simulink model "modelo_BDA"  (R2021b)
settings: Solver=ode3  StartTime=0.0  StopTime=10.0  FixedStep=1e-6  RelTol=1e-3
(part 1 of 4)
settings Model: Creator=Alejandro TeveraRuiz  LastModifiedBy=Alejandro TeveraRuiz

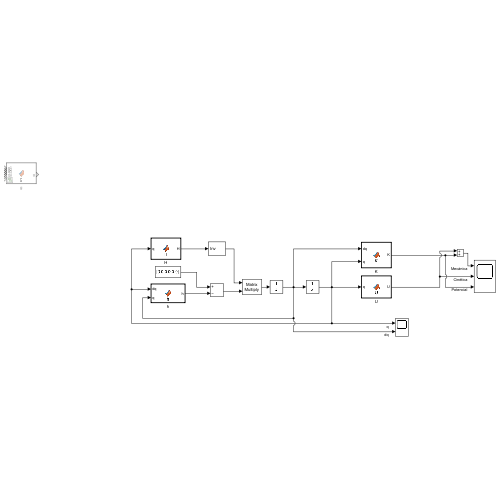
[thumbnail: Simulink's stored preview of the top-level diagram]
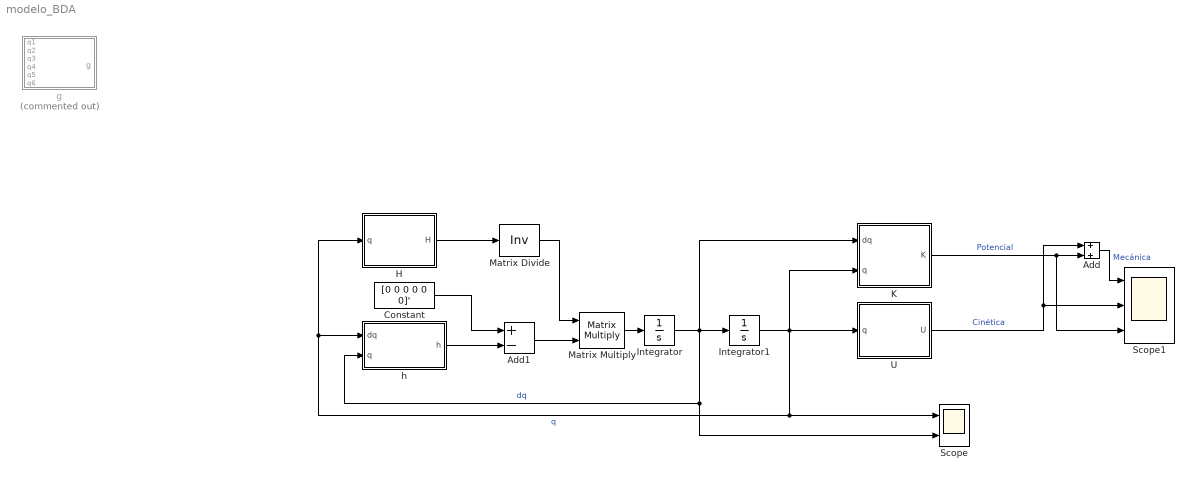
== system modelo_BDA ==
  Add : Sum
  Add1 : Sum  Inputs=+-
  Constant : Constant  Value=[0 0 0 0 0 0]'
  H : MATLAB Function  TreatAsAtomicUnit=on
  Integrator : Integrator  InitialCondition=[0 0 0 0 0 0]'
  Integrator1 : Integrator  InitialCondition=[0 0 0 0 0 0]'
  K : MATLAB Function  TreatAsAtomicUnit=on
  Matrix Divide : Product  Inputs=/  Multiplication=Matrix(*)  OutDataTypeStr=double
  Matrix Multiply : Product  Multiplication=Matrix(*)  OutDataTypeStr=double
  Scope : Scope  NumInputPorts=2
  Scope1 : Scope  NumInputPorts=3
  U : MATLAB Function  TreatAsAtomicUnit=on
  g : MATLAB Function  Commented=on  TreatAsAtomicUnit=on
  h : MATLAB Function  TreatAsAtomicUnit=on
  wires:
  Integrator/1 -> K/1(dq), Scope/2, h/2(q), Integrator1/1  "dq"
  Constant/1 -> Add1/1
  K/1(K) -> Add/2, Scope1/3  "Potencial"
  U/1(U) -> Add/1, Scope1/2  "Cinética"
  Add/1 -> Scope1/1  "Mecánica"
  h/1(h) -> Add1/2
  H/1(H) -> Matrix Divide/1
  Integrator1/1 -> K/2(q), U/1(q), H/1(q), h/1(dq), Scope/1  "q"
  Matrix Multiply/1 -> Integrator/1
  Matrix Divide/1 -> Matrix Multiply/1
  Add1/1 -> Matrix Multiply/2

== matlab function modelo_BDA/H ==
  data: q input; H output
function H = H(q)
%#codegen
q2 = q(2);
q3 = q(3);
q4 = q(4);
q5 = q(5);
q6 = q(6);
%    This function was generated by the Symbolic Math Toolbox version 9.0.
%    01-Dec-2021 19:55:30

t2 = cos(q2);
t3 = cos(q4);
t4 = cos(q5);
t5 = cos(q6);
t6 = sin(q2);
t7 = sin(q4);
t8 = sin(q5);
t9 = sin(q6);
t19 = 9.007199254740992e+15;
t10 = t2.*3.235524933e+1;
t11 = t6.*3.235524933e+1;
t12 = t2.*1.0513390433e+2;
t13 = t6.*1.0513390433e+2;
t14 = t4.*5.110348748545983e-1;
t16 = t8.*5.110348748545983e-1;
t17 = t5.*t8.*4.360410618e+1;
t18 = t8.*t9.*4.360410618e+1;
t20 = t3.*5.157359871151559;
t21 = t4.*t7.*8.595599785252598e-1;
t22 = t3.*t9.*8.595599785252598e-1;
t23 = t7.*t8.*8.595599785252598e-1;
t24 = t3.*t5.*8.595599785252598e-1;
t26 = (q3.*t19)./9.007199254740992e+15;
t29 = q3.*t19.*1.110223024625157e-16i;
t36 = t8.*7.263507131821755e+1;
t37 = t9.*7.263507131821755e+1;
t38 = t5.*1.336375981993753e+2;
t39 = t8.*1.336375981993753e+2;
t42 = t4.*1.356524863046341e+2;
t43 = t3.*3.748034457169395e+1;
t44 = t4.*t9.*1.336375981993753e+2;
t45 = t8.*6.185536839278779e+1;
t46 = t4.*t5.*7.263507131821755e+1;
t47 = t5.*t8.*8.018255891962515e+2;
t50 = t8.*t9.*4.358104279093053e+2;
t51 = t3.*t4.*4.931128922368695e+1;
t52 = t5.*t7.*4.931128922368695e+1;
t53 = t7.*t9.*4.931128922368695e+1;
t54 = t4.*t5.*1.40259874879e-5;
t55 = t4.*t9.*1.40259874879e-5;
t57 = t3.*t8.*t9.*4.931128922368695e+1;
t58 = t5.*t8.*8.415592492740001e-5;
t59 = t8.*t9.*8.415592492740001e-5;
t61 = t3.*t5.*t8.*4.931128922368695e+1;
t71 = t3.*9.473039288601392e+2;
t72 = t7.*9.473039288601392e+2;
t76 = t4.*7.291450524218959e+2;
t77 = t8.*7.291450524218959e+2;
t79 = t5.*1.246862890394724e+3;
t80 = t9.*1.246862890394724e+3;
t82 = t2.*1.908064859676306e+4;
t83 = t8.*6.829347327168682e+1;
t85 = t8.*3.711905458116013e+1;
t86 = t3.*6.892171862305337e+2;
t87 = t8.*4.200920957332826e+3;
t89 = t6.*5.850608528728732e+4;
t90 = t3.*3.746052020548068e+2;
t91 = t3.*5.316839912737671e+1;
t94 = t4.*6.932315136240378e+1;
t95 = t8.*3.161025044569338e+1;
t97 = t4.*t7.*6.243420034246779e+1;
t98 = t3.*t9.*6.243420034246779e+1;
t99 = t5.*t7.*3.583624485303893e+2;
t100 = t7.*t9.*3.583624485303893e+2;
t101 = t4.*2.524704765397172;
t102 = t4.*t5.*(-1.246862890394724e+3);
t103 = t7.*1.451748464558917e+2;
t104 = t4.*t9.*(-1.246862890394724e+3);
t105 = t3.*1.166014482149094e+2;
t106 = t3.*t5.*1.148695310384223e+2;
t107 = t4.*t7.*1.148695310384223e+2;
t109 = t3.*t4.*3.583624485303893e+2;
t110 = t8.*3.603346018435275e-1;
t111 = t4.*t7.*5.316839912737671e+1;
t112 = t7.*5.363537921262857e+2;
t113 = t8.*1.758766552463174e+1;
t114 = t4.*3.603346018435275e-1;
t116 = t5.*3.146556876441599e-4;
t117 = t8.*3.146556876441599e-4;
t118 = t7.*t8.*1.166014482149094e+2;
t119 = t3.*t5.*t8.*3.583624485303893e+2;
t120 = t8.*4.126305645247942e-4;
t121 = t9.*4.126305645247942e-4;
t122 = t3.*t8.*t9.*3.583624485303893e+2;
t124 = t3.*1.607982057580514e-1;
t126 = t3.*t4.*5.363537921262857e+2;
t127 = t3.*t8.*5.363537921262857e+2;
t130 = t4.*t7.*6.060823201364798e-1;
t131 = t4.*t9.*3.146556876441599e-4;
t132 = t7.*t8.*6.060823201364798e-1;
t133 = t4.*t5.*4.126305645247942e-4;
t135 = t3.*t5.*1.205617750389489e-5;
t136 = t3.*t9.*1.205617750389489e-5;
t138 = t8.*5.878411097842592e+2;
t140 = t4.*2.257319383180457e+3;
t144 = t5.*3.383303336574349e+3;
t145 = t9.*1.744166601788531e+3;
t147 = t4.*t5.*1.744166601788531e+3;
t148 = t4.*t9.*3.383303336574349e+3;
t156 = t3.*2.748657914322168e+3;
t164 = t4.*3.726185506152731e+2;
t165 = t8.*3.726185506152731e+2;
t166 = t3.*2.286243086622337e+3;
t167 = t8.*2.14681711570464e+3;
t168 = t7.*6.685860485757689;
t171 = t7.*3.050167960854463e+3;
t172 = t7.*6.689198986080043e+3;
t176 = t3.*t4.*3.581729009555754e+3;
t177 = t7.*t9.*3.581729009555754e+3;
t178 = t4.*t7.*3.610943527871318e+3;
t179 = t4.*t7.*6.267439056015643e+2;
t180 = t3.*t5.*1.071753439291633e+3;
t181 = t7.*t8.*6.267439056015643e+2;
t182 = t3.*t9.*1.071753439291633e+3;
t183 = t3.*t4.*6.589842255968259e+3;
t186 = t5.*t7.*6.589842255968259e+3;
t187 = t7.*3.119613856461354e+4;
t188 = t3.*t4.*3.050167960854463e+3;
t190 = t3.*2.170135173927414;
t192 = t3.*t8.*6.689198986080043e+3;
t193 = t8.*2.108686089031105e-4;
t194 = t8.*8.987910450364716;
t195 = t4.*1.290212183829552;
t196 = t3.*1.511765340066191e+1;
t198 = t3.*t8.*t9.*6.589842255968259e+3;
t201 = t3.*t5.*t8.*3.581729009555754e+3;
t203 = t8.*1.608000299575208e-4;
t204 = t7.*t8.*2.170135173927414;
t205 = t3.*1.454828146091616;
t206 = t7.*1.454828146091616;
t208 = t3.*t4.*3.476976747206118e+1;
t209 = t3.*t8.*3.476976747206118e+1;
t211 = t4.*t7.*1.511765340066191e+1;
t213 = t4.*t7.*3.54680719181798e-4;
t214 = t3.*t9.*3.54680719181798e-4;
t216 = t3.*t5.*2.704654361142649e-4;
t217 = t5.*t7.*6.916395256636513e-4;
t218 = t4.*t7.*2.704654361142649e-4;
t219 = t7.*t9.*6.916395256636513e-4;
t223 = t8.*3.004073079729871e+2;
t224 = t3.*t5.*t8.*6.916395256636513e-4;
t225 = t3.*t8.*t9.*6.916395256636513e-4;
t227 = t4.*1.153568928490484e+3;
t229 = t7.*t8.*1.940301400531246e+3;
t230 = t4.*t7.*5.052846917024227e+2;
t235 = t3.*2.862617746347316e+4;
t249 = t3.*t5.*2.908152143330287e+3;
t250 = t3.*t9.*1.499215806777825e+3;
t15 = -t13;
t25 = -t23;
t27 = cos(t26);
t28 = sin(t26);
t30 = exp(t29);
t31 = -t29;
t48 = -t44;
t49 = -t45;
t56 = t11+t12;
t62 = -t61;
t63 = t16+t21;
t84 = -t77;
t92 = t4.*t79;
t93 = t4.*t80;
t96 = -t90;
t108 = -t94;
t115 = -t110;
t123 = -t114;
t125 = -t116;
t128 = -t119;
t129 = -t121;
t134 = -t130;
t137 = -t136;
t139 = -t138;
t141 = t20+t51;
t161 = -t156;
t169 = -t164;
t189 = -t176;
t191 = -t180;
t197 = -t192;
t199 = -t194;
t200 = -t195;
t202 = -t196;
t207 = -t201;
t210 = -t204;
t215 = -t209;
t221 = -t211;
t222 = -t214;
t226 = -t224;
t228 = -t227;
t253 = -t250;
t275 = t37+t38+4.360410618e+1;
t280 = t18+t36+t55;
t282 = t17+t39+t54;
t303 = t71-8.631091645042425e+1;
t304 = t72+9.559948463095517e-2;
t311 = t101+t113;
t312 = t103+t124;
t443 = t79+t145+4.358104279093053e+2;
t446 = t80+t144+8.018255891962515e+2;
t531 = t187+t205+2.538346896821816;
t532 = t58+t104+t120+t147;
t533 = t59+t102+t117+t148;
t537 = t206+t235-3.371409213983255e+2;
t556 = t47+t50+t87+t131+t133;
t32 = 1.0./t30;
t33 = t3.*t27;
t34 = t7.*t27;
t40 = t30-1.0;
t60 = t10+t15;
t64 = t14+t25;
t66 = t5.*t63.*6.0;
t68 = t9.*t63.*6.0;
t70 = t27.*1.318958611e+1;
t142 = t5.*t63.*4.360410618e+1;
t143 = t9.*t63.*4.360410618e+1;
t150 = t27.*3.811321279694577e+2;
t151 = t27.*3.422984996757468e+1;
t155 = t27.*3.079131064925427e+1;
t170 = t30.*3.694216783411725e-1;
t173 = t30.*1.305783216588275e-1;
t212 = t42+t49;
t220 = t46+t48;
t232 = t9.*t63.*4.358104279093053e+2;
t234 = t5.*t63.*8.018255891962515e+2;
t237 = t5.*t63.*8.415592492740001e-5;
t238 = t9.*t63.*8.415592492740001e-5;
t241 = t3.*t19.*t28.*5.673626844500105e-17;
t242 = t7.*t19.*t28.*5.673626844500105e-17;
t243 = t4.*t19.*t28.*9.543032792050485e-17;
t244 = t8.*t19.*t28.*9.543032792050485e-17;
t245 = t3.*t19.*t28.*3.404176106700063e-16;
t248 = t27.*2.227646919556693e+3;
t252 = t27.*8.579529175625027e+2;
t256 = t27.*2.467380792691235;
t259 = t30.*3.269483204543573;
t264 = t30.*1.334999662191606e+1;
t271 = t27.*1.104616756676389e-4;
t272 = t27.*5.202289239433555e-4;
t285 = t3.*t19.*t28.*2.556183965391409e-15;
t286 = t7.*t19.*t28.*2.556183965391409e-15;
t287 = t19.*t28.*4.869208971920574e-15;
t288 = t7.*t19.*t28.*9.827649182848514e-15;
t289 = t3.*t19.*t28.*2.473934273532809e-15;
t292 = t7.*t19.*t28.*4.958440210927941e-15;
t293 = t7.*t19.*t28.*7.425392937311983e-15;
t295 = t3.*t19.*t28.*7.425392937311983e-15;
t297 = t30.*3.857674212413887e+2;
t299 = t30.*1.091297471081935e+1;
t305 = t30.*4.456000120203464e+1;
t306 = t27.*3.608035586078749e-4;
t313 = t121+t125;
t314 = t116+t129;
t315 = t76+t139;
t316 = t84+t140;
t317 = t8.*t19.*t28.*1.275307981867505e-14;
t318 = t3.*t19.*t28.*4.549259187470966e-14;
t319 = t19.*t28.*1.611764571317528e-14;
t320 = t3.*t19.*t28.*1.117556177536684e-13;
t321 = t7.*t19.*t28.*1.117556177536684e-13;
t323 = t3.*t19.*t28.*2.524584390187751e-13;
t324 = t7.*t19.*t28.*2.524584390187751e-13;
t325 = t7.*t19.*t28.*1.068943235898118e-13;
t326 = t3.*t19.*t28.*7.696415878211547e-15;
t327 = t7.*t19.*t28.*5.39324412732078e-14;
t328 = t4.*t19.*t28.*1.294536125128302e-14;
t330 = t7.*t19.*t28.*9.582436671975919e-15;
t331 = t8.*t19.*t28.*6.931588674426758e-15;
t332 = t3.*t19.*t28.*2.472625742899312e-14;
t335 = t19.*t28.*1.78521870351002e-17;
t338 = t3.*t19.*t28.*3.509442785897641e-15;
t340 = t8.*t19.*t28.*5.90287808936737e-15;
t341 = t3.*t19.*t28.*1.061367489795852e-17;
t342 = t19.*t28.*2.126613508315838e-14;
t345 = t4.*t19.*t28.*6.72886546633755e-17;
t346 = t8.*t19.*t28.*6.72886546633755e-17;
t347 = t19.*t28.*9.790736217417458e-22;
t349 = t19.*t28.*1.646800527103812e-21;
t356 = t30.*2.254739352916933e+3;
t357 = t19.*t28.*t56.*5.673626844500105e-17;
t360 = t30.*2.497388846980927;
t362 = t30.*5.576400544494359e+2;
t365 = t30.*5.642007925493603e-5;
t371 = t30.*2.303752062145191e-4;
t373 = t19.*t28.*6.295748150968656e-14;
t374 = t7.*t19.*t28.*3.067061459005602e-13;
t375 = t7.*t19.*t28.*6.726247428052494e-13;
t376 = t7.*t19.*t28.*6.078928606401748e-13;
t378 = t7.*t19.*t28.*1.333145046183106e-12;
t380 = t4.*t19.*t28.*6.958255145423523e-14;
t381 = t8.*t19.*t28.*4.008952645263927e-13;
t382 = t8.*t19.*t28.*6.958255145423523e-14;
t384 = t3.*t19.*t28.*1.509061667990639e-13;
t385 = t3.*t19.*t28.*1.657497724402608e-13;
t389 = t3.*t19.*t28.*4.691552578623493e-13;
t390 = t3.*t19.*t28.*1.291537270195008e-12;
t391 = t19.*t28.*4.740092871521216e-16;
t392 = t8.*t19.*t28.*1.678396688371765e-15;
t393 = t3.*t19.*t28.*1.432423273139473e-16;
t394 = t3.*t19.*t28.*9.978585125263967e-16;
t395 = t4.*t19.*t28.*2.409334036643134e-16;
t396 = t7.*t19.*t28.*7.599994046755678e-16;
t398 = t3.*t19.*t28.*9.602764472540121e-17;
t399 = t8.*t19.*t28.*3.002769545393412e-20;
t400 = t7.*t19.*t28.*9.602764472540121e-17;
t401 = t7.*t19.*t28.*6.448744418276857e-12;
t402 = t7.*t19.*t28.*3.19687103847679e-12;
t403 = t19.*t28.*4.337843352208199e-20;
t410 = t7.*t19.*t28.*1.670884143038041e-15;
t411 = t8.*t19.*t28.*3.937747008262415e-20;
t416 = t8.*t19.*t28.*5.609786987186535e-14;
t417 = t19.*t28.*3.910962660750154e-13;
t418 = t4.*t19.*t28.*2.154167289582227e-13;
t419 = t19.*t28.*t56.*1.893759423098155e-16;
t423 = t3.*t19.*t28.*3.027237730074418e-12;
t425 = t3.*t19.*t28.*6.279111109874485e-12;
t430 = t30.*2.268539354478371e-4;
t432 = t19.*t28.*2.007862416620223e-13;
t433 = t19.*t28.*2.261065882456945e-13;
t438 = t19.*t28.*5.703946554323684e-14;
t452 = t19.*t28.*t56.*1.74698406676951e-15;
t454 = t19.*t28.*t56.*1.942073956592427e-15;
t459 = t19.*t28.*1.428243658465093e-13;
t491 = t19.*t28.*t56.*5.091700655507849e-16;
t530 = t161+t168+2.094342917444822e+3;
t540 = t91+t123+t126+t132;
t541 = t105+t115+t127+t134;
t585 = t95+t108+t111+t112+t118;
t665 = t166+t188+t192+t199+t200+t204+t221;
t666 = t165+t172+t179+t190+t208+t228+t229;
t667 = t169+t171+t181+t202+t215+t223+t230;
t35 = t34.*6.0;
t41 = t40.^2;
t65 = t5.*t64;
t67 = t9.*t64;
t73 = t34.*4.360410618e+1;
t74 = t33.*2.286892447e+1;
t75 = t34.*2.286892447e+1;
t81 = t33.*6.520967601e+1;
t152 = t34.*4.358104279093053e+2;
t153 = t33.*1.328674864713371e+3;
t154 = t34.*1.328674864713371e+3;
t157 = t34.*8.018255891962515e+2;
t158 = t34.*6.185536839278779e+1;
t159 = t33.*1.688943762888624e+2;
t160 = t34.*1.356524863046341e+2;
t163 = t33.*7.092789006718835e+2;
t174 = t34.*1.870703729528352e-1;
t175 = t32.*3.694216783411725e-1;
t184 = t32.*1.305783216588275e-1;
t246 = -t242;
t247 = -t243;
t251 = t34.*4.522154679359383e+3;
t254 = t34.*2.65978307941329e+3;
t255 = t34.*2.92140771649329e+3;
t257 = t33.*4.033568532372886e+3;
t258 = t33.*8.84585468187615e+3;
t261 = t33.*9.245169992678717;
t262 = t32.*3.269483204543573;
t263 = t34.*2.524704765397172;
t266 = t33.*4.153012702745543e+4;
t267 = t34.*1.758766552463174e+1;
t268 = t32.*1.334999662191606e+1;
t269 = t33.*1.692526621106363;
t270 = t34.*1.692526621106363;
t274 = -t271;
t276 = -t272;
t277 = t34.*3.854027039691565e+4;
t294 = -t288;
t296 = -t293;
t298 = t34.*2.310978750639558e+3;
t300 = t32.*3.857674212413887e+2;
t301 = t32.*1.091297471081935e+1;
t302 = t33.*4.724604290218056;
t307 = t32.*4.456000120203464e+1;
t308 = -t306;
t322 = -t318;
t329 = -t321;
t333 = -t324;
t334 = -t325;
t336 = -t327;
t337 = -t328;
t339 = -t330;
t343 = -t341;
t344 = t34+t241;
t350 = -t347;
t358 = t32.*2.254739352916933e+3;
t359 = t19.*t28.*t60.*9.543032792050485e-17;
t363 = t32.*2.497388846980927;
t364 = t32.*5.576400544494359e+2;
t366 = t32.*5.642007925493603e-5;
t368 = t52+t57+t66;
t369 = t53+t62+t68;
t372 = t32.*2.303752062145191e-4;
t377 = -t373;
t379 = -t374;
t383 = -t376;
t386 = -t378;
t387 = -t380;
t388 = -t382;
t397 = -t393;
t404 = -t396;
t405 = -t398;
t406 = -t399;
t407 = -t400;
t408 = -t401;
t409 = -t402;
t412 = -t403;
t413 = -t410;
t420 = -t418;
t421 = t19.*t28.*t60.*3.18530082611956e-16;
t424 = -t423;
t427 = -t425;
t431 = t32.*2.268539354478371e-4;
t434 = -t432;
t439 = -t438;
t455 = -t452;
t457 = t19.*t28.*t60.*2.938424872360468e-15;
t461 = t19.*t28.*t60.*3.266565807075334e-15;
t493 = -t491;
t497 = t19.*t28.*t60.*8.564233717611997e-16;
t589 = t19.*t28.*t530.*9.543032792050485e-17;
t69 = -t65;
t78 = -t74;
t88 = -t81;
t146 = t24+t67;
t162 = -t157;
t185 = -t174;
t231 = t67.*1.336375981993753e+2;
t233 = t65.*7.263507131821755e+1;
t239 = t65.*1.40259874879e-5;
t240 = t67.*1.40259874879e-5;
t260 = -t258;
t265 = -t263;
t273 = -t270;
t278 = -t277;
t279 = t65.*1.246862890394724e+3;
t281 = t67.*1.246862890394724e+3;
t290 = t65.*4.126305645247942e-4;
t291 = t67.*3.146556876441599e-4;
t309 = t65.*1.744166601788531e+3;
t310 = t67.*3.383303336574349e+3;
t348 = t33+t246;
t351 = t5.*t344;
t352 = t9.*t344;
t361 = -t359;
t367 = t32.*t41.*5.499266393288274;
t370 = t32.*t41.*7.936984065608979;
t414 = t4.*t344.*4.234075154e+1;
t415 = t8.*t344.*4.234075154e+1;
t422 = -t421;
t426 = t32.*t41.*1.589092398552061e+2;
t428 = t32.*t41.*1.835560892149977e+1;
t429 = t32.*t41.*2.649229280878313e+1;
t435 = t32.*t41.*t56.*2.196325630278387e-1;
t436 = t32.*t41.*t60.*2.196325630278387e-1;
t440 = t4.*t344.*3.077051043151931e+2;
t441 = t37.*t344;
t442 = t38.*t344;
t448 = t4.*t344.*4.605359747732407e+2;
t450 = t8.*t344.*4.605359747732407e+2;
t465 = -t461;
t466 = t32.*t41.*9.287951675407251e+2;
t467 = t32.*t41.*1.02874981515943;
t468 = t32.*t41.*4.326292055563303e+2;
t469 = t32.*t41.*1.369651538214088e-4;
t470 = t32.*t41.*9.489849812415379e-5;
t471 = t32.*t41.*t56.*6.34659991754557;
t472 = t32.*t41.*t56.*7.330958613472507e-1;
t473 = t32.*t41.*t60.*7.330958613472507e-1;
t475 = t4.*t344.*5.658316341762099e+3;
t476 = t4.*t344.*3.07542350777483e+3;
t477 = t4.*t344.*2.619002784534197e+3;
t478 = t4.*t344.*4.465233410425356e+3;
t479 = t8.*t344.*5.743628218407764e+3;
t480 = t79.*t344;
t482 = t80.*t344;
t486 = t4.*t344.*2.985478799712556e+1;
t487 = t8.*t344.*2.985478799712556e+1;
t494 = t121.*t344;
t495 = t116.*t344;
t506 = t170+t175+2.61156643317655e-1;
t507 = t173+t184+7.38843356682345e-1;
t508 = t32.*t41.*1.515649212522415e-4;
t509 = t32.*t41.*t56.*3.709470474531108e+1;
t510 = t32.*t41.*t56.*7.517989680436807;
t511 = t32.*t41.*t56.*4.108674547820486e-2;
t512 = t32.*t41.*t60.*6.762774476882097;
t514 = t144.*t344;
t515 = t145.*t344;
t516 = t32.*t41.*t56.*3.790105603165286e-6;
t518 = t32.*t41.*t60.*3.790105603165286e-6;
t520 = t32.*t41.*t56.*3.25782309086522e-6;
t521 = t32.*t41.*t60.*1.936876142599284e-6;
t542 = t311.*t344;
t599 = t344.*t537;
t691 = t344.*t665;
t149 = t22+t69;
t236 = -t233;
t283 = -t279;
t284 = -t281;
t353 = t4.*t348;
H = ft_1({t100,t106,t107,t109,t122,t128,t135,t137,t141,t142,t143,t146,t149,t150,t151,t152,t153,t154,t155,t157,t158,t159,t160,t162,t163,t166,t167,t177,t178,t182,t183,t185,t186,t188,t189,t19,t191,t193,t194,t195,t197,t198,t2,t203,t207,t210,t211,t212,t213,t216,t217,t218,t219,t222,t225,t226,t231,t232,t234,t236,t237,t238,t239,t240,t243,t244,t245,t247,t248,t249,t251,t252,t253,t254,t255,t256,t257,t258,t259,t260,t261,t262,t263,t264,t265,t266,t267,t268,t269,t27,t273,t274,t275,t276,t278,t28,t280,t282,t283,t284,t285,t286,t287,t289,t290,t291,t292,t294,t295,t296,t297,t298,t299,t3,t300,t301,t302,t303,t304,t305,t307,t308,t309,t310,t311,t312,t313,t314,t315,t316,t317,t318,t319,t320,t322,t323,t326,t329,t331,t332,t333,t334,t335,t336,t337,t338,t339,t340,t342,t343,t344,t345,t346,t348,t349,t35,t350,t351,t352,t353,t356,t357,t358,t36,t360,t361,t362,t363,t364,t365,t366,t367,t368,t369,t37,t370,t371,t372,t375,t377,t378,t379,t38,t381,t382,t383,t384,t385,t386,t387,t388,t389,t39,t390,t391,t392,t393,t394,t395,t397,t399,t4,t404,t405,t406,t407,t408,t409,t411,t412,t413,t414,t415,t416,t417,t418,t419,t42,t420,t422,t424,t426,t427,t428,t429,t43,t430,t431,t433,t434,t435,t436,t439,t44,t440,t441,t442,t443,t446,t448,t45,t450,t454,t455,t457,t459,t46,t465,t466,t467,t468,t469,t470,t471,t472,t473,t475,t476,t477,t478,t479,t480,t482,t486,t487,t493,t494,t497,t5,t506,t507,t508,t509,t51,t510,t511,t512,t514,t515,t516,t518,t520,t521,t530,t531,t532,t533,t537,t540,t541,t542,t556,t56,t585,t589,t599,t6,t60,t63,t64,t65,t665,t666,t667,t67,t691,t7,t70,t73,t74,t75,t76,t77,t78,t79,t8,t80,t81,t82,t83,t85,t86,t88,t89,t9,t96,t97,t98,t99});
end
function H = ft_1(ct)
t100 = ct{1};
t106 = ct{2};
t107 = ct{3};
t109 = ct{4};
t122 = ct{5};
t128 = ct{6};
t135 = ct{7};
t137 = ct{8};
t141 = ct{9};
t142 = ct{10};
t143 = ct{11};
t146 = ct{12};
t149 = ct{13};
t150 = ct{14};
t151 = ct{15};
t152 = ct{16};
t153 = ct{17};
t154 = ct{18};
t155 = ct{19};
t157 = ct{20};
t158 = ct{21};
t159 = ct{22};
t160 = ct{23};
t162 = ct{24};
t163 = ct{25};
t166 = ct{26};
t167 = ct{27};
t177 = ct{28};
t178 = ct{29};
t182 = ct{30};
t183 = ct{31};
t185 = ct{32};
t186 = ct{33};
t188 = ct{34};
t189 = ct{35};
t19 = ct{36};
t191 = ct{37};
t193 = ct{38};
t194 = ct{39};
t195 = ct{40};
t197 = ct{41};
t198 = ct{42};
t2 = ct{43};
t203 = ct{44};
t207 = ct{45};
t210 = ct{46};
t211 = ct{47};
t212 = ct{48};
t213 = ct{49};
t216 = ct{50};
t217 = ct{51};
t218 = ct{52};
t219 = ct{53};
t222 = ct{54};
t225 = ct{55};
t226 = ct{56};
t231 = ct{57};
t232 = ct{58};
t234 = ct{59};
t236 = ct{60};
t237 = ct{61};
t238 = ct{62};
t239 = ct{63};
t240 = ct{64};
t243 = ct{65};
t244 = ct{66};
t245 = ct{67};
t247 = ct{68};
t248 = ct{69};
t249 = ct{70};
t251 = ct{71};
t252 = ct{72};
t253 = ct{73};
t254 = ct{74};
t255 = ct{75};
t256 = ct{76};
t257 = ct{77};
t258 = ct{78};
t259 = ct{79};
t260 = ct{80};
t261 = ct{81};
t262 = ct{82};
t263 = ct{83};
t264 = ct{84};
t265 = ct{85};
t266 = ct{86};
t267 = ct{87};
t268 = ct{88};
t269 = ct{89};
t27 = ct{90};
t273 = ct{91};
t274 = ct{92};
t275 = ct{93};
t276 = ct{94};
t278 = ct{95};
t28 = ct{96};
t280 = ct{97};
t282 = ct{98};
t283 = ct{99};
t284 = ct{100};
t285 = ct{101};
t286 = ct{102};
t287 = ct{103};
t289 = ct{104};
t290 = ct{105};
t291 = ct{106};
t292 = ct{107};
t294 = ct{108};
t295 = ct{109};
t296 = ct{110};
t297 = ct{111};
t298 = ct{112};
t299 = ct{113};
t3 = ct{114};
t300 = ct{115};
t301 = ct{116};
t302 = ct{117};
t303 = ct{118};
t304 = ct{119};
t305 = ct{120};
t307 = ct{121};
t308 = ct{122};
t309 = ct{123};
t310 = ct{124};
t311 = ct{125};
t312 = ct{126};
t313 = ct{127};
t314 = ct{128};
t315 = ct{129};
t316 = ct{130};
t317 = ct{131};
t318 = ct{132};
t319 = ct{133};
t320 = ct{134};
t322 = ct{135};
t323 = ct{136};
t326 = ct{137};
t329 = ct{138};
t331 = ct{139};
t332 = ct{140};
t333 = ct{141};
t334 = ct{142};
t335 = ct{143};
t336 = ct{144};
t337 = ct{145};
t338 = ct{146};
t339 = ct{147};
t340 = ct{148};
t342 = ct{149};
t343 = ct{150};
t344 = ct{151};
t345 = ct{152};
t346 = ct{153};
t348 = ct{154};
t349 = ct{155};
t35 = ct{156};
t350 = ct{157};
t351 = ct{158};
t352 = ct{159};
t353 = ct{160};
t356 = ct{161};
t357 = ct{162};
t358 = ct{163};
t36 = ct{164};
t360 = ct{165};
t361 = ct{166};
t362 = ct{167};
t363 = ct{168};
t364 = ct{169};
t365 = ct{170};
t366 = ct{171};
t367 = ct{172};
t368 = ct{173};
t369 = ct{174};
t37 = ct{175};
t370 = ct{176};
t371 = ct{177};
t372 = ct{178};
t375 = ct{179};
t377 = ct{180};
t378 = ct{181};
t379 = ct{182};
t38 = ct{183};
t381 = ct{184};
t382 = ct{185};
t383 = ct{186};
t384 = ct{187};
t385 = ct{188};
t386 = ct{189};
t387 = ct{190};
t388 = ct{191};
t389 = ct{192};
t39 = ct{193};
t390 = ct{194};
t391 = ct{195};
t392 = ct{196};
t393 = ct{197};
t394 = ct{198};
t395 = ct{199};
t397 = ct{200};
t399 = ct{201};
t4 = ct{202};
t404 = ct{203};
t405 = ct{204};
t406 = ct{205};
t407 = ct{206};
t408 = ct{207};
t409 = ct{208};
t411 = ct{209};
t412 = ct{210};
t413 = ct{211};
t414 = ct{212};
t415 = ct{213};
t416 = ct{214};
t417 = ct{215};
t418 = ct{216};
t419 = ct{217};
t42 = ct{218};
t420 = ct{219};
t422 = ct{220};
t424 = ct{221};
t426 = ct{222};
t427 = ct{223};
t428 = ct{224};
t429 = ct{225};
t43 = ct{226};
t430 = ct{227};
t431 = ct{228};
t433 = ct{229};
t434 = ct{230};
t435 = ct{231};
t436 = ct{232};
t439 = ct{233};
t44 = ct{234};
t440 = ct{235};
t441 = ct{236};
t442 = ct{237};
t443 = ct{238};
t446 = ct{239};
t448 = ct{240};
t45 = ct{241};
t450 = ct{242};
t454 = ct{243};
t455 = ct{244};
t457 = ct{245};
t459 = ct{246};
t46 = ct{247};
t465 = ct{248};
t466 = ct{249};
t467 = ct{250};
t468 = ct{251};
t469 = ct{252};
t470 = ct{253};
t471 = ct{254};
t472 = ct{255};
t473 = ct{256};
t475 = ct{257};
t476 = ct{258};
t477 = ct{259};
t478 = ct{260};
t479 = ct{261};
t480 = ct{262};
t482 = ct{263};
t486 = ct{264};
t487 = ct{265};
t493 = ct{266};
t494 = ct{267};
t497 = ct{268};
t5 = ct{269};
t506 = ct{270};
t507 = ct{271};
t508 = ct{272};
t509 = ct{273};
t51 = ct{274};
t510 = ct{275};
t511 = ct{276};
t512 = ct{277};
t514 = ct{278};
t515 = ct{279};
t516 = ct{280};
t518 = ct{281};
t520 = ct{282};
t521 = ct{283};
t530 = ct{284};
t531 = ct{285};
t532 = ct{286};
t533 = ct{287};
t537 = ct{288};
t540 = ct{289};
t541 = ct{290};
t542 = ct{291};
t556 = ct{292};
t56 = ct{293};
t585 = ct{294};
t589 = ct{295};
t599 = ct{296};
t6 = ct{297};
t60 = ct{298};
t63 = ct{299};
t64 = ct{300};
t65 = ct{301};
t665 = ct{302};
t666 = ct{303};
t667 = ct{304};
t67 = ct{305};
t691 = ct{306};
t7 = ct{307};
t70 = ct{308};
t73 = ct{309};
t74 = ct{310};
t75 = ct{311};
t76 = ct{312};
t77 = ct{313};
t78 = ct{314};
t79 = ct{315};
t8 = ct{316};
t80 = ct{317};
t81 = ct{318};
t82 = ct{319};
t83 = ct{320};
t85 = ct{321};
t86 = ct{322};
t88 = ct{323};
t89 = ct{324};
t9 = ct{325};
t96 = ct{326};
t97 = ct{327};
t98 = ct{328};
t99 = ct{329};
t354 = t8.*t348;
t355 = -t352;
t437 = -t436;
t444 = t352.*4.358104279093053e+2;
t447 = t351.*8.018255891962515e+2;
t460 = t351.*1.40259874879e-5;
t462 = t352.*1.40259874879e-5;
t474 = -t473;
t481 = -t475;
t483 = t76.*t348;
t484 = t77.*t348;
t485 = t352.*(-1.246862890394724e+3);
t490 = -t486;
t501 = t351.*(-3.146556876441599e-4);
t513 = -t512;
t517 = t351.*(-3.383303336574349e+3);
t519 = -t518;
t522 = -t521;
t534 = t56.*t507;
t535 = t60.*t506;
t598 = t348.*t531;
t600 = -t599;
t601 = t287+t357+t361;
t604 = t259+t262+t370+1.849951749091285e+1;
t607 = t264+t268+t367+9.437562846167879;
t634 = t342+t419+t422;
t639 = t85+t97+t100+t128+t135+t143+t240;
t640 = t83+t99+t107+t122+t137+t142+t239;
t689 = t155+t299+t301+t349+t429+6.174821949234504e+1;
t690 = t151+t305+t307+t350+t428+3.150096765411469e+1;
t692 = -t691;
t695 = t252+t362+t364+t412+t468+8.92670750207894e+2;
t703 = t276+t365+t366+t433+t469+3.192382947754238e-4;
t704 = t274+t371+t372+t434+t470+1.628600027717729e-4;
t739 = t150+t159+t185+t297+t300+t339+t343+t426+2.727120002407305e+2;
t742 = t167+t177+t178+t186+t198+t207+t216+t222+t232+t234+t290+t291;
t445 = t353.*7.263507131821755e+1;
t449 = t353.*1.336375981993753e+2;
t451 = t354.*1.356524863046341e+2;
t453 = t353.*6.185536839278779e+1;
t456 = t353.*7.051076542399408e-1;
t458 = t354.*7.051076542399408e-1;
t464 = -t460;
t488 = t353.*(-7.291450524218959e+2);
t489 = t353.*4.200920957332826e+3;
t492 = t354.*2.524704765397172;
t498 = t353.*1.758766552463174e+1;
t499 = t353.*4.126305645247942e-4;
t500 = t353.*3.146556876441599e-4;
t503 = t353.*5.878411097842592e+2;
t504 = t354.*2.257319383180457e+3;
t523 = t244+t353;
t524 = t247+t354;
t525 = -t5.*(t243-t354);
t527 = -t9.*(t243-t354);
t536 = -t535;
t543 = t534.*3.33782865;
t544 = t535.*2.889644336e+1;
t545 = t535.*3.33782865;
t548 = t5.*(t243-t354).*(-7.263507131821755e+1);
t551 = t9.*(t243-t354).*(-1.336375981993753e+2);
t552 = t5.*(t243-t354).*(-4.358104279093053e+2);
t553 = t5.*(t243-t354).*7.263507131821755e+1;
t554 = t9.*(t243-t354).*(-8.018255891962515e+2);
t555 = t5.*(t243-t354).*4.358104279093053e+2;
t557 = t9.*(t243-t354).*(-1.40259874879e-5);
t560 = t5.*(t243-t354).*(-1.40259874879e-5);
t561 = t9.*(t243-t354).*1.40259874879e-5;
t563 = t5.*(t243-t354).*1.40259874879e-5;
t564 = t535.*1.688943762888624e+2;
t565 = t534.*3.079131064925427e+1;
t567 = t535.*3.422984996757468e+1;
t569 = -t79.*(t243-t354);
t570 = -t80.*(t243-t354);
t571 = t535.*1.870703729528352e-1;
t572 = t5.*(t243-t354).*1.246862890394724e+3;
t574 = t534.*1.72565741205e-5;
t575 = t535.*1.72565741205e-5;
t577 = t5.*(t243-t354).*(-4.126305645247942e-4);
t578 = t9.*(t243-t354).*(-3.146556876441599e-4);
t579 = t5.*(t243-t354).*4.126305645247942e-4;
t580 = t9.*(t243-t354).*3.146556876441599e-4;
t581 = t5.*(t243-t354).*(-1.744166601788531e+3);
t582 = t9.*(t243-t354).*(-3.383303336574349e+3);
t583 = t5.*(t243-t354).*1.744166601788531e+3;
t584 = t9.*(t243-t354).*3.383303336574349e+3;
t586 = t534.*8.818711196088817e-6;
t587 = t535.*1.483306048043653e-5;
t594 = -t316.*(t243-t354);
t595 = t316.*(t243-t354);
t602 = t7.*t601;
t603 = t3.*t601;
t605 = t3.*t604;
t606 = t7.*t604;
t608 = t43+t98+t106+t109+t231+t236;
t635 = t70+t607;
t656 = -t443.*(t352+t5.*(t243-t354));
t657 = t443.*(t352+t5.*(t243-t354));
t686 = -t532.*(t352+t5.*(t243-t354));
t688 = t532.*(t352+t5.*(t243-t354));
t696 = -t666.*(t243-t354);
t698 = t437+t534+t604;
t708 = t27.*t695;
t736 = t19.*t28.*t703.*9.543032792050485e-17;
t737 = t19.*t28.*t704.*5.673626844500105e-17;
t740 = t86+t182+t183+t203+t218+t219+t226+t238+t249+t283+t310;
t741 = t96+t189+t191+t193+t213+t217+t225+t237+t253+t284+t309;
t463 = -t458;
t496 = -t492;
t502 = -t500;
t505 = -t504;
t526 = t5.*t523.*6.0;
t528 = t9.*t523.*6.0;
t538 = t5.*t523.*4.360410618e+1;
t539 = t9.*t523.*4.360410618e+1;
t546 = -t544;
t547 = t9.*t523.*4.358104279093053e+2;
t549 = -t545;
t550 = t5.*t523.*8.018255891962515e+2;
t558 = t5.*t523.*8.415592492740001e-5;
t559 = t9.*t523.*8.415592492740001e-5;
t566 = -t564;
t568 = -t567;
t573 = -t571;
t576 = -t575;
t588 = -t587;
t590 = t314.*t523;
t591 = t315.*t523;
t596 = t351+t527;
t597 = t355+t525;
t609 = t603.*2.889644336e+1;
t610 = t602.*2.889644336e+1;
t611 = t602.*1.087689656e+1;
t614 = t605.*2.889644336e+1;
t615 = t606.*2.889644336e+1;
t616 = t605.*1.087689656e+1;
t617 = t603.*6.678442840618982e+2;
t618 = t602.*6.678442840618982e+2;
t621 = t602.*6.185536839278779e+1;
t622 = t603.*1.688943762888624e+2;
t623 = t602.*1.356524863046341e+2;
t625 = t602.*1.870703729528352e-1;
t627 = t605.*6.678442840618982e+2;
t628 = t606.*6.678442840618982e+2;
t629 = t605.*1.356524863046341e+2;
t630 = t606.*1.688943762888624e+2;
t632 = t605.*6.185536839278779e+1;
t633 = t605.*1.870703729528352e-1;
t636 = t4.*t635;
t637 = t8.*t635;
t646 = t36.*t635;
t647 = t39.*t635;
t649 = t42.*t635;
t650 = t45.*t635;
t654 = t523.*t556;
t658 = t75+t295+t606;
t659 = t81+t294+t605;
t660 = t74+t296+t605;
t697 = t523.*t667;
t699 = t3.*t698;
t700 = t7.*t698;
t701 = t435+t536+t607;
t717 = t435+t536+t635;
t738 = -t737;
t743 = t474+t543+t689;
t760 = t523.*t742;
t764 = -t741.*(t352+t5.*(t243-t354));
t765 = t741.*(t352+t5.*(t243-t354));
t799 = t454+t465+t519+t574+t703;
t529 = -t526;
t562 = -t559;
t592 = -t590;
t593 = -t591;
t612 = -t610;
t613 = -t611;
t619 = -t617;
t620 = -t618;
t624 = -t621;
t626 = -t625;
t631 = -t628;
t638 = -t637;
t641 = t637.*7.26735103;
t643 = t636.*1.087689656e+1;
t644 = t637.*1.087689656e+1;
t648 = t637.*(-7.263507131821755e+1);
t651 = t637.*(-6.185536839278779e+1);
t652 = t637.*7.051076542399408e-1;
t653 = t636.*7.051076542399408e-1;
t655 = t446.*t596;
t661 = t4.*t658;
t662 = t8.*t658;
t663 = t5.*t659;
t664 = t9.*t659;
t675 = t38.*t659;
t677 = t37.*t659;
t685 = t533.*t596;
t693 = t154+t319+t323+t615;
t694 = t153+t333+t335+t614;
t702 = -t699;
t705 = t699.*2.889644336e+1;
t706 = t700.*2.889644336e+1;
t707 = t699.*1.087689656e+1;
t709 = t699.*6.678442840618982e+2;
t710 = t700.*6.678442840618982e+2;
t711 = t699.*1.356524863046341e+2;
t712 = t700.*1.688943762888624e+2;
t714 = t699.*6.185536839278779e+1;
t716 = t699.*1.870703729528352e-1;
t718 = t4.*t717;
t719 = t8.*t717;
t726 = t39.*t717;
t727 = t36.*t717;
t730 = t45.*t717;
t731 = t42.*t717;
t744 = t472+t549+t690;
t759 = t163+t334+t337+t340+t451+t453+t616;
t762 = t596.*t740;
t766 = t75+t285+t603+t700;
t771 = -t5.*(t81-t292-t602+t699);
t772 = -t9.*(t81-t292-t602+t699);
t773 = t9.*(t81-t292-t602+t699);
t778 = t5.*(t81-t292-t602+t699).*(-7.26735103);
t780 = t5.*(t81-t292-t602+t699).*7.26735103;
t787 = t5.*(t81-t292-t602+t699).*(-1.336375981993753e+2);
t789 = t38.*(t81-t292-t602+t699);
t790 = t37.*(t81-t292-t602+t699);
t791 = t5.*(t81-t292-t602+t699).*(-1.40259874879e-5);
t793 = t5.*(t81-t292-t602+t699).*1.40259874879e-5;
t794 = t471+t546+t739;
t795 = t251+t261+t390+t413+t417+t630+t633;
t800 = t455+t457+t516+t576+t704;
t801 = t248+t266+t273+t356+t358+t391+t405+t408+t466+t627+1.593951290590465e+3;
t805 = t19.*t28.*t799.*9.543032792050485e-17;
t808 = t510+t513+t565+t568+t695;
t642 = -t641;
t645 = -t644;
t668 = t661.*7.26735103;
t669 = t663.*7.26735103;
t670 = t664.*7.26735103;
t671 = t661.*1.087689656e+1;
t672 = t662.*1.087689656e+1;
t673 = t661.*7.263507131821755e+1;
t674 = t661.*1.336375981993753e+2;
t678 = t662.*1.356524863046341e+2;
t679 = t661.*6.185536839278779e+1;
t680 = t661.*7.051076542399408e-1;
t681 = t662.*7.051076542399408e-1;
t683 = t663.*1.40259874879e-5;
t684 = t664.*1.40259874879e-5;
t687 = -t685;
t713 = -t710;
t715 = -t711;
t720 = -t719;
t721 = t719.*7.26735103;
t723 = t718.*1.087689656e+1;
t724 = t719.*1.087689656e+1;
t728 = t719.*(-1.336375981993753e+2);
t729 = t719.*(-7.263507131821755e+1);
t732 = t719.*(-6.185536839278779e+1);
t733 = t718.*7.051076542399408e-1;
t734 = t719.*7.051076542399408e-1;
t745 = t415+t636+t662;
t746 = t414+t638+t661;
t763 = -t762;
t767 = t4.*t766;
t768 = t8.*t766;
t769 = t78+t286+t602+t702;
t770 = t88+t292+t602+t702;
t777 = t773.*(-7.26735103);
t779 = t773.*7.26735103;
t788 = t773.*(-7.263507131821755e+1);
t792 = t773.*(-1.40259874879e-5);
t796 = t154+t319+t320+t609+t706;
t797 = t153+t329+t335+t612+t705;
t798 = t19.*t28.*t795.*9.543032792050485e-17;
t802 = t256+t269+t278+t360+t363+t377+t407+t427+t467+t631+1.765488401398446;
t806 = t19.*t28.*t800.*5.673626844500105e-17;
t809 = t27.*t808;
t810 = t348.*t801;
t815 = t163+t336+t337+t340+t451+t453+t613+t707;
t838 = t248+t266+t273+t356+t358+t391+t405+t409+t466+t509+t566+t620+t709+1.593951290590465e+3;
t843 = t251+t261+t389+t404+t417+t622+t626+t712+t716;
t676 = -t674;
t682 = -t680;
t722 = -t721;
t725 = -t724;
t735 = -t734;
t747 = t5.*t745;
t748 = t9.*t745;
t761 = t35+t245+t746;
t774 = t767.*7.26735103;
t775 = t767.*1.087689656e+1;
t776 = t768.*1.087689656e+1;
t781 = t767.*1.336375981993753e+2;
t782 = t767.*7.263507131821755e+1;
t783 = t767.*6.185536839278779e+1;
t784 = t768.*1.356524863046341e+2;
t785 = t767.*7.051076542399408e-1;
t786 = t768.*7.051076542399408e-1;
t803 = t160+t326+t346+t450+t456+t643+t672;
t804 = t158+t338+t345+t448+t463+t645+t671;
t807 = -t806;
t811 = t344.*t802;
t816 = t73+t289+t440+t441+t442+t551+t553+t642+t668;
t817 = t415+t718+t768;
t818 = t414+t720+t767;
t834 = t257+t267+t383+t387+t394+t416+t484+t487+t503+t632+t653+t681;
t839 = t256+t269+t278+t360+t363+t377+t407+t424+t467+t511+t573+t619+t713+1.765488401398446;
t841 = (t243-t354).*(t260+t263+t378+t388+t393+t418-t483+t486+t505-t629-t652+t680);
t842 = t348.*t838;
t846 = t19.*t28.*t843.*9.543032792050485e-17;
t848 = t254+t384+t392+t395+t477+t479+t496+t498+t649+t651+t678+t679;
t749 = -t748;
t750 = t747.*7.26735103;
t751 = t748.*7.26735103;
t753 = t747.*7.263507131821755e+1;
t754 = t748.*1.336375981993753e+2;
t756 = t747.*1.40259874879e-5;
t757 = t748.*1.40259874879e-5;
t812 = -t811;
t813 = t528+t664+t747;
t819 = t5.*t817;
t820 = t9.*t817;
t831 = t35+t245+t818;
t835 = t258+t265+t382+t386+t397+t420+t483+t490+t504+t629+t652+t682;
t836 = t160+t326+t346+t450+t456+t723+t776;
t837 = t158+t338+t345+t448+t463+t725+t775;
t840 = t523.*t834;
t844 = t344.*t839;
t847 = t73+t289+t440+t441+t442+t551+t553+t722+t774;
t849 = t344.*t848;
t856 = t257+t267+t379+t387+t394+t416+t484+t487+t503+t624+t714+t733+t786;
t857 = t260+t263+t375+t388+t393+t418+t486+t488+t505+t623+t715+t735+t785;
t867 = t254+t384+t392+t395+t477+t479+t496+t498+t731+t732+t783+t784;
t752 = -t751;
t755 = -t754;
t758 = -t757;
t814 = t526+t663+t749;
t821 = t819.*7.26735103;
t822 = t820.*7.26735103;
t824 = t820.*1.336375981993753e+2;
t825 = t819.*7.263507131821755e+1;
t827 = t819.*1.40259874879e-5;
t828 = t820.*1.40259874879e-5;
t833 = t331+t445+t464+t539+t561+t670+t750;
t845 = -t844;
t850 = t529+t771+t820;
t851 = t528+t773+t819;
t855 = t162+t322+t399+t481+t485+t500+t517+t559+t569+t584+t647+t676+t684+t756;
t858 = t523.*t856;
t859 = -t857.*(t243-t354);
t860 = t857.*(t243-t354);
t861 = -t596.*(t157+t318+t406+t475+t482+t502+t514+t562+t572+t582-t637.*1.336375981993753e+2+t674-t684-t756);
t863 = t596.*(t157+t318+t406+t475+t482+t502+t514+t562+t572+t582-t637.*1.336375981993753e+2+t674-t684-t756);
t868 = t344.*t867;
t823 = -t822;
t826 = -t824;
t829 = -t827;
t830 = -t828;
t832 = t317+t449+t462+t538+t563+t669+t752;
t853 = t331+t445+t464+t539+t561+t779+t821;
t854 = t152+t332+t411+t476+t480+t499+t515+t558+t570+t583+t648+t673+t683+t758;
t865 = t381+t489+t494+t501+t547+t550+t579+t580+t675+t677+t753+t755;
t852 = t317+t449+t462+t538+t563+t780+t823;
t862 = -t854.*(t352+t5.*(t243-t354));
t864 = t854.*(t352+t5.*(t243-t354));
t866 = t523.*t865;
t869 = t157+t318+t406+t475+t482+t502+t514+t562+t572+t582+t728+t781+t792+t829;
t870 = t152+t332+t411+t476+t480+t499+t515+t558+t570+t583+t729+t782+t793+t830;
t874 = t381+t489+t494+t501+t547+t550+t579+t580+t789+t790+t825+t826;
t871 = t596.*t869;
t872 = -t870.*(t352+t5.*(t243-t354));
t873 = t870.*(t352+t5.*(t243-t354));
t875 = t523.*t874;
et1 = t82+t89+t805+t807+t809+t842+t845+t846+t858+t860+t868+t871+t873+t875+t852.*(t526-t820+t5.*(t81-t292-t602+t699))+t601.*t634+t698.*t743+t701.*t744+t717.*t794+t766.*t796+t817.*t836+t818.*t837+t831.*t847+t851.*t853;
et2 = t56.*(t2.*2.143246204038348e+3+t6.*6.595899367493489e+2+3.22231575312482e+2);
et3 = -t60.*(t2.*(-6.595899367493489e+2)+t6.*2.143246204038348e+3+4.573234736449676e+2);
et4 = t797.*(t74-t286-t602+t699)+t815.*(t81-t292-t602+t699)+2.531266629412227e+5;
et5 = t298+t302+t308+t430+t431+t459+t493+t497+t508+t520+t522+t586+t588-t602.*9.559948463095517e-2;
et6 = t603.*8.631091645042425e+1+t699.*9.559948463095517e-2;
et7 = t700.*8.631091645042425e+1-t3.*t796.*1.291687373922119e+1;
et8 = t7.*t797.*1.291687373922119e+1+t7.*t815.*4.931128922368695e+1+t3.*t839.*8.595599785252598e-1;
et9 = t7.*t838.*8.595599785252598e-1-t3.*t867.*8.595599785252598e-1+t63.*t856+t64.*t857+t63.*t874-t141.*t847-t146.*t869-t149.*t870+t368.*t852+t369.*t853;
et10 = t3.*t19.*t28.*2.397546984890625e-13;
et11 = t7.*t19.*t28.*(-3.88386200657948e-16);
et12 = t3.*t4.*t837.*(-4.931128922368695e+1)-t3.*t8.*t836.*4.931128922368695e+1;
et13 = 3.03129842504483e-4;
et14 = t708+t736+t738+t798+t810+t812+t840+t841+t849+t863+t864+t866+t604.*t689+t607.*t690+t658.*t693+t660.*t694+t635.*t739+t659.*t759+t745.*t803+t746.*t804+t761.*t816+t813.*t833+t814.*t832;
et15 = t28.^2.*8.400913676692644e+3;
et16 = 1.896531265228407e+4;
et17 = t298+t302+t308+t430+t431+t459+t508+t605.*9.559948463095517e-2;
et18 = t606.*8.631091645042425e+1-t146.*(t157+t318+t406+t475+t482+t502+t514+t562+t572+t582-t637.*1.336375981993753e+2+t674-t684-t756);
et19 = t3.*t693.*(-1.291687373922119e+1)+t7.*t694.*1.291687373922119e+1;
et20 = t7.*t759.*4.931128922368695e+1+t3.*t802.*8.595599785252598e-1+t7.*t801.*8.595599785252598e-1-t3.*t848.*8.595599785252598e-1+t63.*t834+t63.*t865-t141.*t816-t149.*t854+t368.*t832;
et21 = t369.*t833+t64.*(t260+t263+t378+t388+t393+t418-t483+t486+t505-t629-t652+t680);
et22 = t3.*t19.*t28.*6.600205872441553e-13;
et23 = t7.*t19.*t28.*(-8.538800689339779e-16);
et24 = t3.*t4.*t804.*(-4.931128922368695e+1)-t3.*t8.*t803.*4.931128922368695e+1;
et25 = 3.03129842504483e-4;
et26 = t255+t385+t392+t395+t444+t447+t478+t479+t496+t498+t554+t555-t637.*1.054594745727878e+2+t649+t661.*1.054594745727878e+2+t678;
et27 = t5.*(t157+t318+t406+t475+t482+t502+t514+t562+t572+t582-t637.*1.336375981993753e+2+t674-t684-t756)+t9.*t854;
et28 = t308+t430+t431+t439+t493+t497+t508+t520+t522+t586+t588+t589+t598+t600+t692+t696+t697+t760+t763+t765+t640.*(t526-t820+t5.*(t81-t292-t602+t699))+t312.*t717-t303.*t766-t540.*t818-t541.*t817-t608.*t831+t639.*t851+t304.*(t74-t286-t602+t699)+t585.*(t81-t292-t602+t699);
et29 = 3.03129842504483e-4;
et30 = t308+t430+t431+t439+t508+t589+t598+t600+t692+t696+t697+t760+t763+t765+t312.*t635-t303.*t658+t304.*t660+t585.*t659-t540.*t746-t541.*t745-t608.*t761+t639.*t813+t640.*t814;
et31 = 3.03129842504483e-4;
et32 = t3.*(-1.40466005326373e+3);
et33 = t7.*3.416707876634484;
et34 = t3.*t303.*1.291687373922119e+1+t7.*t304.*1.291687373922119e+1+t7.*t531.*8.595599785252598e-1;
et35 = t3.*t537.*8.595599785252598e-1+t51.*t540+t7.*t585.*4.931128922368695e+1+t3.*t665.*8.595599785252598e-1+t63.*t667-t64.*t666+t141.*t608+t63.*t742+t146.*t740-t149.*t741+t368.*t640+t369.*t639;
et36 = t3.*t8.*t541.*4.931128922368695e+1;
et37 = 1.288118518170248e+3;
et38 = t3.*(-2.5111251540525e+3)+t65.*4.358104279093053e+2;
et39 = t67.*(-8.018255891962515e+2)+t194+t195+t197+t210+t211-t3.*t4.*5.200342652036798e+3;
et40 = t3.*t5.*(-6.892171862305337e+2)-t3.*t9.*3.746052020548068e+2-t5.*t740;
et41 = t9.*t741;
et42 = t530-t7.*t212.*4.931128922368695e+1-t3.*t311.*8.595599785252598e-1-t63.*t315+t64.*t316+t63.*t556+t280.*t369+t282.*t368+t146.*t533-t149.*t532+t141.*(t44-t46);
et43 = t3.*t4.^2.*(-3.476976747206118e+1);
et44 = t3.*t8.^2.*(-3.476976747206118e+1);
et45 = t5.*8.018255891962515e+2+t9.*4.358104279093053e+2+t5.*t446+t9.*t443;
et46 = 2.92140771649329e+3;
mt1 = [et1+et2+et3+et4,t82+t89+t708+t736+t738+t798+t810+t812+t840+t841+t849+t863+t864+t866+t832.*(t526-t820+t5.*(t81-t292-t602+t699))+t342.*t601+t689.*t698+t690.*t701+t717.*t739+t693.*t766+t803.*t817+t804.*t818+t816.*t831+t833.*t851+t694.*(t74-t286-t602+t699)+t759.*(t81-t292-t602+t699)+1.896531265228407e+4,et28+et29];
mt2 = [t542+t593+t595+t654+t687+t688+t843+t282.*(t526-t820+t5.*(t81-t292-t602+t699))+t4.*t818.*7.051076542399408e-1+t8.*t817.*7.051076542399408e-1+t280.*t851-t831.*(t44-t46)-t212.*(t81-t292-t602+t699)];
mt3 = [t592+t655+t657+t867+t9.*(t526-t820+t5.*(t81-t292-t602+t699)).*1.40259874879e-5-t5.*t851.*1.40259874879e-5+t275.*t831,t874];
mt4 = [t82+t89+t805+t807+t809+t842+t845+t846+t858+t860+t868+t871+t873+t875+t287.*t634+t604.*t743+t607.*t744+t635.*t794+t658.*t796+t660.*t797+t659.*t815+t745.*t836+t746.*t837+t761.*t847+t813.*t853+t814.*t852+1.896531265228407e+4,et14+et15+et16,et30+et31];
mt5 = [t542+t593+t595+t654+t687+t688+t795+t4.*t746.*7.051076542399408e-1+t8.*t745.*7.051076542399408e-1-t212.*t659+t280.*t813+t282.*t814-t761.*(t44-t46)];
mt6 = [t592+t655+t657+t848-t5.*t813.*1.40259874879e-5+t9.*t814.*1.40259874879e-5+t275.*t761,t865,et5+et6+et7+et8+et9+et10+et11+et12+et13,et17+et18+et19+et20+et21+et22+et23+et24+et25,et32+et33+et34+et35+et36+et37,et42+et43+et44];
mt7 = [-t166-t188+t194+t195+t197+t210+t211-t5.*t369.*1.40259874879e-5+t9.*t368.*1.40259874879e-5-t63.*t314-t141.*t275-t146.*t446-t149.*t443,t742];
mt8 = [t843+t4.*t857+t8.*t856+t8.*t874+t5.*t8.*t852.*6.0+t8.*t9.*t853.*6.0+t4.*t5.*t870-t4.*t9.*t869,t795+t8.*t834+t8.*t865+t4.*(t260+t263+t378+t388+t393+t418-t483+t486+t505-t629-t652+t680)-t4.*t9.*(t157+t318+t406+t475+t482+t502+t514+t562+t572+t582-t637.*1.336375981993753e+2+t674-t684-t756)+t5.*t8.*t832.*6.0+t8.*t9.*t833.*6.0+t4.*t5.*t854,t530-t4.*t666+t8.*t667+t8.*t742+t5.*t8.*t640.*6.0+t8.*t9.*t639.*6.0+t4.*t5.*t741+t4.*t9.*t740];
mt9 = [t4.*t316-t8.*t315+t8.*t556+t5.*t8.*t282.*6.0+t8.*t9.*t280.*6.0+t4.*t5.*t532+t4.*t9.*t533+4.098238731829628e+3,t311-t8.*t314+t4.*t5.*t443-t4.*t9.*t446,t556];
mt10 = [t255+t385+t392+t395+t444+t447+t478+t479+t496+t498+t554+t555-t719.*1.054594745727878e+2+t731+t767.*1.054594745727878e+2+t784+t5.*t869+t9.*t870,et26+et27,et38+et39+et40+et41];
mt11 = [t311+t4.*t5.*4.358104279093053e+2-t4.*t9.*8.018255891962515e+2-t5.*t533+t9.*t532,et45+et46,t313,t874,t865,t742,t556,t313];
mt12 = [4.200920957332826e+3];
H = real(reshape([mt1,mt2,mt3,mt4,mt5,mt6,mt7,mt8,mt9,mt10,mt11,mt12],6,6));
end
